simulink model "PIDcontroller"  (R2016a)
settings: Solver=ode4  StartTime=0.0  StopTime=10.0  FixedStep=0.01  RelTol=1e-3
settings Model: Creator=ikuma  LastModifiedBy=ikuma

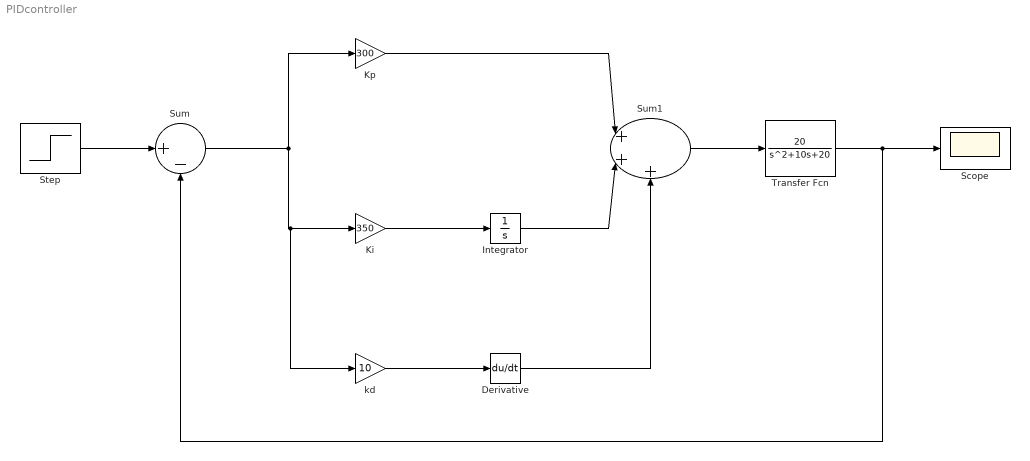
== system PIDcontroller ==
  Derivative : Derivative
  Integrator : Integrator
  Ki : Gain  Gain=350
  Kp : Gain  Gain=300
  Scope : Scope
  Step : Step  Time=0  SampleTime=0
  Sum : Sum  Inputs=|+-
  Sum1 : Sum  Inputs=|+++
  Transfer Fcn : TransferFcn  Numerator=[20]  Denominator=[1 10 20]
  kd : Gain  Gain=10
  wires:
  Sum1/1 -> Transfer Fcn/1
  Transfer Fcn/1 -> Sum/2, Scope/1
  Sum/1 -> Kp/1, kd/1, Ki/1
  Step/1 -> Sum/1
  Ki/1 -> Integrator/1
  kd/1 -> Derivative/1
  Kp/1 -> Sum1/1
  Integrator/1 -> Sum1/2
  Derivative/1 -> Sum1/3
